simulink model "controller"  (R2024b)
settings: Solver=FixedStepAuto  StartTime=0.0  StopTime=100  FixedStep=1/10  RelTol=1e-3  EnableMultiTasking=on
undefined symbols (not defined in the file): MAX_RDB_ENGAGE_SPEED, MAX_TORQUE, MAX_TORQUE_REVERSE
libraries: arduinolib x15
settings Model: ExtModeTrigDuration=2  Creator=DAUIN-Win10  LastModifiedBy=aayan
settings SolverCC: AutoInsertRateTranBlk=on
settings OptimizationCC: EnhancedBackFolding=on  PassReuseOutputArgsAs=Individual arguments  ZeroExternalMemoryAtStartup=off  ZeroInternalMemoryAtStartup=off  MaxStackSize=64  OptimizeBlockOrder=speed  DifferentSizesBufferReuse=on  OptimizationCustomize=off  EfficientTunableParamExpr=on
settings DebuggingCC: ParameterTunabilityLossMsg=error  UnconnectedInputMsg=warning  UnconnectedOutputMsg=warning  UnconnectedLineMsg=warning
settings HardwareCC: ProdBitPerInt=16  ProdBitPerPointer=16  ProdBitPerSizeT=16  ProdBitPerPtrDiffT=16  ProdLargestAtomicFloat=None  ProdWordSize=8  ProdHWDeviceType=Atmel->AVR
settings ModelReferenceCC: EnableRefExpFcnMdlSchedulingChecks=on
settings SFSimCC: MATLABDynamicMemAlloc=off
settings RTWCC: Description=Embedded Coder  SystemTargetFile=ert.tlc  HardwareBoard=Arduino Uno  TemplateMakefile=ert_default_tmf  GenerateReport=on  Toolchain=Arduino AVR  BuildConfiguration=Faster Runs  GPUComputeCapability=3.5  DLArmComputeVersion=19.05
settings CodeAppCC: ForceParamTrailComments=on  IgnoreCustomStorageClasses=off  OperatorAnnotations=on  SimulinkDataObjDesc=on  SFDataObjDesc=on  InsertBlockDesc=on
settings ERTTargetCC: SupportVariableSizeSignals=on  ExtModeTransport=3  ExtModeStaticAlloc=on  ExtModeAutomaticAllocSize=off  ExtModeStaticAllocSize=250  ExtModeMexFile=ext_xcp  ExtModeIntrfLevel=Level2 - Open  InlinedParameterPlacement=Hierarchical

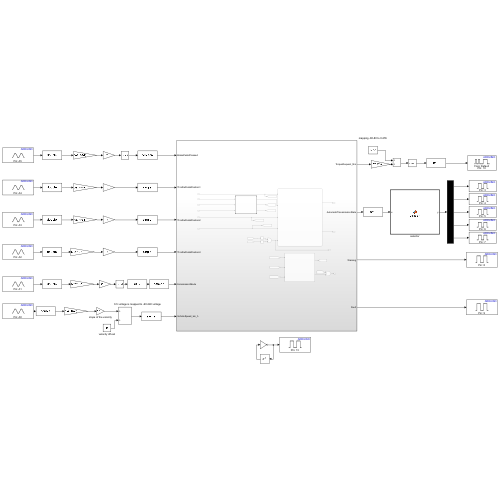
[thumbnail: Simulink's stored preview of the top-level diagram]
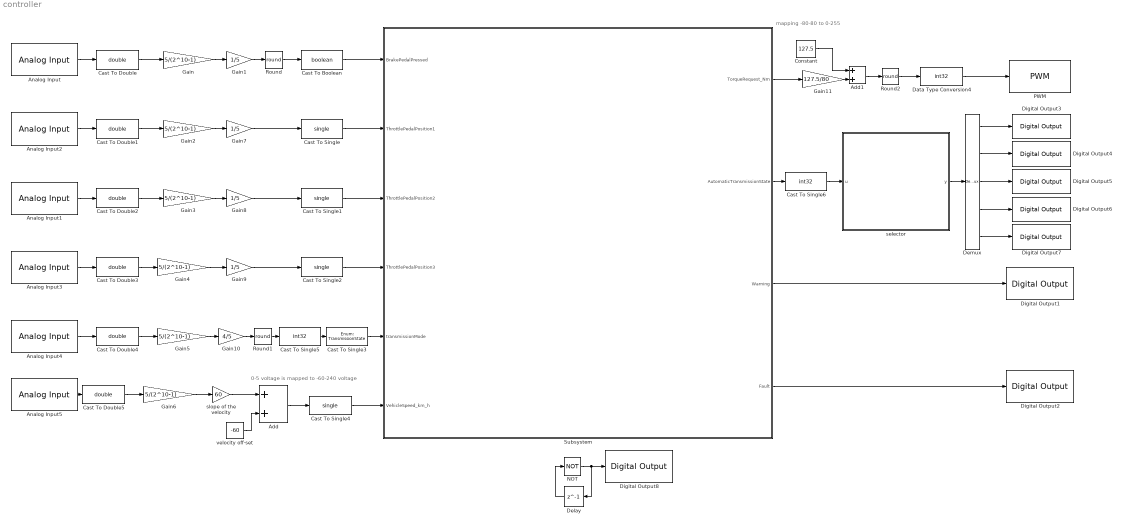
== system controller ==
  note: mapping -80-80 to 0-255
  note: 0-5 voltage is mapped to -60-240 voltage
  Add : Sum
  Add1 : Sum
  Analog Input : arduinolib/Analog Input  pinNumber=5  ReadResultsOnly=off  ConversionTriggerSource=Software  ExternalTriggerType=uint32( 0 )  OutputDataType=uint16  EnableConversionCompleteNotify=off  EnableOuputStatus=off  SampleTime=-1  blockPlatform=arduino
      settings: SourceProductName=Common
  Analog Input1 : arduinolib/Analog Input  pinNumber=3  ReadResultsOnly=off  ConversionTriggerSource=Software  ExternalTriggerType=uint32( 0 )  OutputDataType=uint16  EnableConversionCompleteNotify=off  EnableOuputStatus=off  SampleTime=-1  blockPlatform=arduino
      settings: SourceProductName=Common
  Analog Input2 : arduinolib/Analog Input  pinNumber=4  ReadResultsOnly=off  ConversionTriggerSource=Software  ExternalTriggerType=uint32( 0 )  OutputDataType=uint16  EnableConversionCompleteNotify=off  EnableOuputStatus=off  SampleTime=-1  blockPlatform=arduino
      settings: SourceProductName=Common
  Analog Input3 : arduinolib/Analog Input  pinNumber=2  ReadResultsOnly=off  ConversionTriggerSource=Software  ExternalTriggerType=uint32( 0 )  OutputDataType=uint16  EnableConversionCompleteNotify=off  EnableOuputStatus=off  SampleTime=-1  blockPlatform=arduino
      settings: SourceProductName=Common
  Analog Input4 : arduinolib/Analog Input  pinNumber=1  ReadResultsOnly=off  ConversionTriggerSource=Software  ExternalTriggerType=uint32( 0 )  OutputDataType=uint16  EnableConversionCompleteNotify=off  EnableOuputStatus=off  SampleTime=-1  blockPlatform=arduino
      settings: SourceProductName=Common
  Analog Input5 : arduinolib/Analog Input  pinNumber=0  ReadResultsOnly=off  ConversionTriggerSource=Software  ExternalTriggerType=uint32( 0 )  OutputDataType=uint16  EnableConversionCompleteNotify=off  EnableOuputStatus=off  SampleTime=-1  blockPlatform=arduino
      settings: SourceProductName=Common
  Cast To Boolean : DataTypeConversion  OutDataTypeStr=boolean  SaturateOnIntegerOverflow=off  RndMeth=Floor
  Cast To Double{,1..5} (6 alike) : DataTypeConversion  OutDataTypeStr=double  SaturateOnIntegerOverflow=off  RndMeth=Floor
  Cast To Single{,1..2,4} (4 alike) : DataTypeConversion  OutDataTypeStr=single  SaturateOnIntegerOverflow=off  RndMeth=Floor
  Cast To Single3 : DataTypeConversion  OutDataTypeStr=Enum: TransmissionState  SaturateOnIntegerOverflow=off  RndMeth=Floor
  Cast To Single5 : DataTypeConversion  OutDataTypeStr=int32  SaturateOnIntegerOverflow=off  RndMeth=Floor
  Cast To Single6 : DataTypeConversion  OutDataTypeStr=int32  SaturateOnIntegerOverflow=off  RndMeth=Floor
  Constant : Constant  Value=127.5
  Data Type Conversion4 : DataTypeConversion  OutDataTypeStr=int32  SaturateOnIntegerOverflow=off  RndMeth=Floor
  Delay : Delay  DelayLength=1  InputProcessing=Columns as channels (frame based)
  Demux : Demux  Outputs=5
  Digital Output1 : arduinolib/Digital Output  pinNumber=8  Direction=output  blockPlatform=arduino
      settings: SourceProductName=Common
  Digital Output2 : arduinolib/Digital Output  pinNumber=9  Direction=output  blockPlatform=arduino
      settings: SourceProductName=Common
  Digital Output3 : arduinolib/Digital Output  pinNumber=3  Direction=output  blockPlatform=arduino
      settings: SourceProductName=Common
  Digital Output4 : arduinolib/Digital Output  pinNumber=4  Direction=output  blockPlatform=arduino
      settings: SourceProductName=Common
  Digital Output5 : arduinolib/Digital Output  pinNumber=5  Direction=output  blockPlatform=arduino
      settings: SourceProductName=Common
  Digital Output6 : arduinolib/Digital Output  pinNumber=6  Direction=output  blockPlatform=arduino
      settings: SourceProductName=Common
  Digital Output7 : arduinolib/Digital Output  pinNumber=7  Direction=output  blockPlatform=arduino
      settings: SourceProductName=Common
  Digital Output8 : arduinolib/Digital Output  pinNumber=13  Direction=output  blockPlatform=arduino
      settings: SourceProductName=Common
  Gain{,2..6} (6 alike) : Gain  Gain=5/(2^10-1)
  Gain{1,7..9} (4 alike) : Gain  Gain=1/5
  Gain10 : Gain  Gain=4/5
  Gain11 : Gain  Gain=127.5/80
  NOT : Logic  Operator=NOT  IconShape=distinctive  AllPortsSameDT=off  OutDataTypeStr=boolean
  PWM : arduinolib/PWM  pinNumber=10  frequencyType=Default  desiredFrequency=490.2  achievableFrequency=490.2
      settings: SourceProductName=Common
  Round : Rounding  Operator=round
  Round1 : Rounding  Operator=round
  Round2 : Rounding  Operator=round
  Subsystem : Subsystem
  selector : MATLAB Function  TreatAsAtomicUnit=on
  slope of the velocity : Gain  Gain=60
  velocity off-set : Constant  Value=-60
  wires:
  Analog Input/1 -> Cast To Double/1
  Analog Input2/1 -> Cast To Double1/1
  Analog Input5/1 -> Cast To Double5/1
  Analog Input4/1 -> Cast To Double4/1
  Analog Input3/1 -> Cast To Double3/1
  Analog Input1/1 -> Cast To Double2/1
  Subsystem/1(TorqueRequest_Nm) -> Gain11/1
  Subsystem/2(AutomaticTransmissionState) -> Cast To Single6/1
  Cast To Double/1 -> Gain/1
  Gain/1 -> Gain1/1
  Gain1/1 -> Round/1
  Round/1 -> Cast To Boolean/1
  Cast To Boolean/1 -> Subsystem/1(BrakePedalPressed)
  Cast To Double1/1 -> Gain2/1
  Cast To Double2/1 -> Gain3/1
  Cast To Double3/1 -> Gain4/1
  Cast To Double4/1 -> Gain5/1
  Cast To Double5/1 -> Gain6/1
  Gain2/1 -> Gain7/1
  Gain3/1 -> Gain8/1
  Gain4/1 -> Gain9/1
  Gain5/1 -> Gain10/1
  Gain6/1 -> slope of the velocity/1
  Gain7/1 -> Cast To Single/1
  Gain8/1 -> Cast To Single1/1
  Gain9/1 -> Cast To Single2/1
  Gain10/1 -> Round1/1
  Cast To Single/1 -> Subsystem/2(ThrottlePedalPosition1)
  Cast To Single1/1 -> Subsystem/3(ThrottlePedalPosition2)
  Cast To Single2/1 -> Subsystem/4(ThrottlePedalPosition3)
  slope of the velocity/1 -> Add/1
  velocity off-set/1 -> Add/2
  Add/1 -> Cast To Single4/1
  Cast To Single3/1 -> Subsystem/5(transmissionMode)
  Cast To Single4/1 -> Subsystem/6(VehicleSpeed_km_h)
  Demux/1 -> Digital Output3/1
  Demux/2 -> Digital Output4/1
  Demux/3 -> Digital Output5/1
  Demux/4 -> Digital Output6/1
  Demux/5 -> Digital Output7/1
  Subsystem/3(Warning) -> Digital Output1/1
  Subsystem/4(Fault) -> Digital Output2/1
  Constant/1 -> Add1/1
  Gain11/1 -> Add1/2
  Add1/1 -> Round2/1
  selector/1(y) -> Demux/1
  Round2/1 -> Data Type Conversion4/1
  Data Type Conversion4/1 -> PWM/1
  Round1/1 -> Cast To Single5/1
  Cast To Single5/1 -> Cast To Single3/1
  Cast To Single6/1 -> selector/1(u)
  NOT/1 -> Digital Output8/1, Delay/1
  Delay/1 -> NOT/1

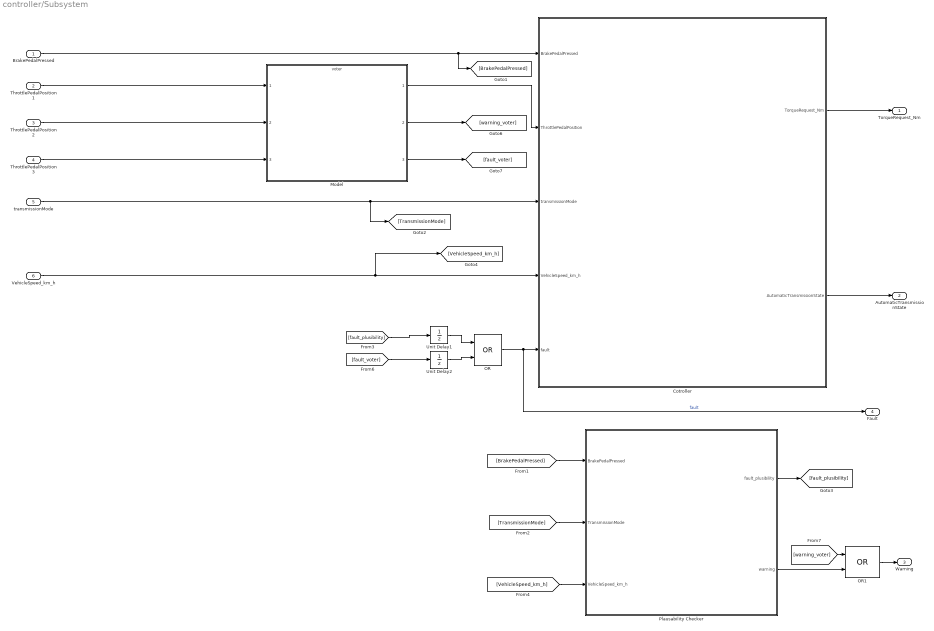
== system controller/Subsystem ==
  BrakePedalPressed : Inport
  ThrottlePedalPosition1 : Inport  Port=2
  ThrottlePedalPosition2 : Inport  Port=3
  ThrottlePedalPosition3 : Inport  Port=4
  transmissionMode : Inport  Port=5
  VehicleSpeed_km_h : Inport  Port=6
  Cotroller : Stateflow chart  TreatAsAtomicUnit=on
      settings: PortSchema="{\"entries\":[{\"content\":{\"sides\":[{\"content\":{\"connectorIds\":[\"In1\",\"In2\",\"In3\",\"In4\",\"In5\"]},\"type\":\"ConnectorPlacement.EquallySpacedRectSide\",\"uuid\":\"fa3865f3-071a-4523-b56b-dfcb7b7ff1e1\"},{\"content\":{\"connectorIds\":[\"Out2\",\"Out1\"],\"side\":\"RIGHT\"},\"type\":\"ConnectorPlacement.EquallySpacedRectSide\",\"uuid\":\"97edfdd5-6ca1-4319-83ef-4a85a5b2efa4\"},{\"content\":{\"side\":\"TOP\"},\"type\":\"ConnectorPlacement.EquallySpacedRectSide\",\"uuid\":\"bfa350c0-61e1-4051-a5a1-0c01bc7888ec\"}]},\"type\":\"ConnectorPlacement.EquallySpacedConnector\",\"uuid\":\"0069708a-38e0-4c12-a9eb-137e78633e28\"}],\"packageUris\":[\"http://schema.mathworks.com/mf0/Connector/R2020b\"],\"version\":\"1.0\"}"
  Model : ModelReference  ModelNameDialog=voter.slx  SimulationMode=Normal  ModelReferenceVersion=1.26
  OR : Logic  Operator=OR  IconShape=distinctive  AllPortsSameDT=off  OutDataTypeStr=boolean
  OR1 : Logic  Operator=OR  IconShape=distinctive  AllPortsSameDT=off  OutDataTypeStr=boolean
  Plausability Checker : Subsystem
  Unit Delay1 : UnitDelay  SampleTime=-1  HasFrameUpgradeWarning=on
  Unit Delay2 : UnitDelay  SampleTime=-1  HasFrameUpgradeWarning=on
  TorqueRequest_Nm : Outport  OutDataTypeStr=single  Unit=N*m
  AutomaticTransmissionState : Outport  Port=2  OutDataTypeStr=Enum: TransmissionState
  Warning : Outport  Port=3  OutDataTypeStr=boolean
  Fault : Outport  Port=4  OutDataTypeStr=boolean
  wires:
  BrakePedalPressed/1 -> [BrakePedalPressed], Cotroller/1(BrakePedalPressed)
  ThrottlePedalPosition1/1 -> Model/1
  ThrottlePedalPosition3/1 -> Model/3
  ThrottlePedalPosition2/1 -> Model/2
  transmissionMode/1 -> [TransmissionMode], Cotroller/3(transmissionMode)
  Model/2 -> [warning_voter]
  Plausability Checker/2(warning) -> OR1/2
  Model/3 -> [fault_voter]
  Unit Delay2/1 -> OR/2
  OR1/1 -> Warning/1
  Cotroller/1(AutomaticTransmissionState) -> AutomaticTransmissionState/1
  Unit Delay1/1 -> OR/1
  Cotroller/2(TorqueRequest_Nm) -> TorqueRequest_Nm/1
  [fault_plusibility] -> Unit Delay1/1
  [BrakePedalPressed] -> Plausability Checker/1(BrakePedalPressed)
  Plausability Checker/1(fault_plusibility) -> [fault_plusibility]
  [VehicleSpeed_km_h] -> Plausability Checker/3(VehicleSpeed_km_h)
  [fault_voter] -> Unit Delay2/1
  [warning_voter] -> OR1/1
  [TransmissionMode] -> Plausability Checker/2(TransmissionMode)
  VehicleSpeed_km_h/1 -> [VehicleSpeed_km_h], Cotroller/4(VehicleSpeed_km_h)
  Model/1 -> Cotroller/2(ThrottlePedalPosition)
  OR/1 -> Fault/1, Cotroller/5(fault)  "fault"

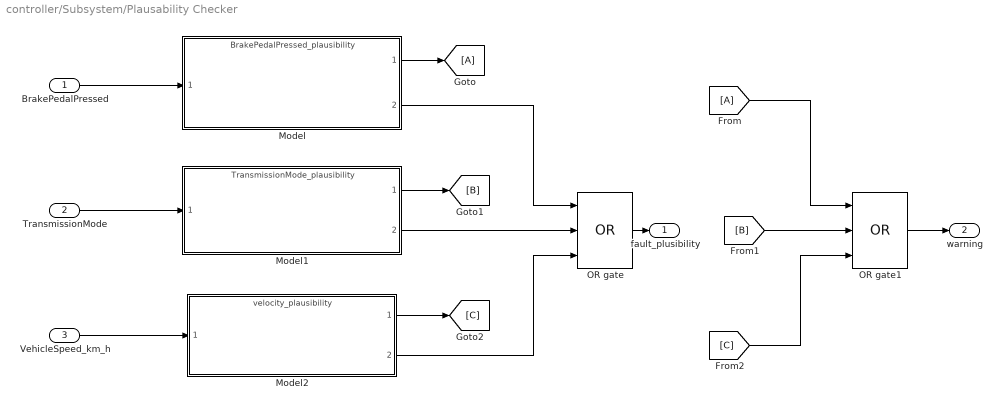
== system controller/Subsystem/Plausability Checker ==
  BrakePedalPressed : Inport
  TransmissionMode : Inport  Port=2  OutDataTypeStr=Enum: TransmissionState
  VehicleSpeed_km_h : Inport  Port=3
  From : From
  Goto : Goto
  Model : ModelReference  ModelNameDialog=BrakePedalPressed_plausibility.slx  SimulationMode=Normal  ModelReferenceVersion=1.19
  Model1 : ModelReference  ModelNameDialog=TransmissionMode_plausibility.slx  SimulationMode=Normal  ModelReferenceVersion=1.13
  Model2 : ModelReference  ModelNameDialog=velocity_plausibility.slx  SimulationMode=Normal  ModelReferenceVersion=1.14
  OR gate : Logic  Operator=OR  Inputs=3  IconShape=distinctive  AllPortsSameDT=off  OutDataTypeStr=boolean
  OR gate1 : Logic  Operator=OR  Inputs=3  IconShape=distinctive  AllPortsSameDT=off  OutDataTypeStr=boolean
  fault_plusibility : Outport  OutDataTypeStr=boolean
  warning : Outport  Port=2
  wires:
  BrakePedalPressed/1 -> Model/1
  Model/1 -> Goto/1
  TransmissionMode/1 -> Model1/1
  Model1/1 -> [B]
  Model/2 -> OR gate/1
  Model1/2 -> OR gate/2
  Model2/2 -> OR gate/3
  OR gate1/1 -> warning/1
  Model2/1 -> [C]
  From/1 -> OR gate1/1
  [B] -> OR gate1/2
  [C] -> OR gate1/3
  OR gate/1 -> fault_plusibility/1
  VehicleSpeed_km_h/1 -> Model2/1

== matlab function controller/selector ==
  data: u input; y output
function y = selector(u)

y = false(1, 5);

if u >= 0 && u <= 4
    y(u+1) = true;
end

== stateflow chart controller/Subsystem/Cotroller ==
  settings: updateMethod=DISCRETE  sampleTime=0.1
  state Park
    en:
    AutomaticTransmissionState = TransmissionState.Park;
    du:
    TorqueRequest_Nm = single(0);
  state Neutral
    en:
    AutomaticTransmissionState = TransmissionState.Neutral;
    du:
    TorqueRequest_Nm = single(0);
  state Drive
    en:
    AutomaticTransmissionState = TransmissionState.Drive;
    state ZeroTorque1
      du:
      TorqueRequest_Nm = single(0);
    state Acceleration
      du:
      TorqueRequest_Nm = single(MAX_TORQUE*(ThrottlePedalPosition));
    state StartToMove
      du:
      TorqueRequest_Nm = single(5);
    (default) -> ZeroTorque1
    ZeroTorque1 -> (junction 99) [order 1] : [BrakePedalPressed ~= 1 && VehicleSpeed_km_h  < 5 ]
    (junction 99) -> StartToMove
    (junction 94) -> ZeroTorque1
    StartToMove -> (junction 94) [order 2] : [BrakePedalPressed == 1]
    ZeroTorque1 -> Acceleration [order 2] : [(BrakePedalPressed ~= 1)]
    Acceleration -> ZeroTorque1 : [ (BrakePedalPressed == 1)]
    StartToMove -> Acceleration [order 1] : [ThrottlePedalPosition > 0 && BrakePedalPressed ~= 1]
  state Brake
    en:
    AutomaticTransmissionState = TransmissionState.Brake
    state AccelerationRegion
      du:
      TorqueRequest_Nm = single(MAX_TORQUE*(3/2)*(ThrottlePedalPosition - (1/3)));
    state ZeroTorque
      TorqueRequest_Nm = single(0);
    state DecelerationRegion
      du:
      TorqueRequest_Nm = single(-MAX_TORQUE*(1 - 3*ThrottlePedalPosition));
    (default) -> AccelerationRegion
    Brake.ZeroTorque -> AccelerationRegion : [ThrottlePedalPosition > (1/3) && BrakePedalPressed == 0]
    AccelerationRegion -> Brake.ZeroTorque [order 2] : [BrakePedalPressed == 1]
    DecelerationRegion -> AccelerationRegion [order 1] : [ (ThrottlePedalPosition >(1/3)) && BrakePedalPressed == 0]
    AccelerationRegion -> DecelerationRegion [order 1] : [ ThrottlePedalPosition < (1/3) && BrakePedalPressed == 0]
    (junction 43) -> Brake.ZeroTorque
    DecelerationRegion -> (junction 43) [order 2] : [VehicleSpeed_km_h < MAX_RDB_ENGAGE_SPEED || BrakePedalPressed == 1]
  state Reverse
    en:
    AutomaticTransmissionState = TransmissionState.Reverse;
    state Deceleration
      du:
      TorqueRequest_Nm = single(-MAX_TORQUE_REVERSE*(ThrottlePedalPosition));
    state ZeroTorque
      TorqueRequest_Nm = single(0);
    (default) -> Deceleration
    Reverse.ZeroTorque -> Deceleration : [(BrakePedalPressed == 0)]
    Deceleration -> Reverse.ZeroTorque : [(BrakePedalPressed == 1)]
  (default) -> Park
  Neutral -> Drive [order 1] : [(BrakePedalPressed == 1) && (VehicleSpeed_km_h > -5) && ((transmissionMode == TransmissionState.Drive) || (transmissionMode == TransmissionState.Brake)) && fault == 0]
  Park -> Neutral : [(BrakePedalPressed == 1) && (transmissionMode ~= TransmissionState.Park) || fault == 1]
  Drive -> Brake [order 1] : [ThrottlePedalPosition > (1/3) && (transmissionMode == TransmissionState.Brake) && fault == 0]
  Brake -> Drive : [ transmissionMode ~= TransmissionState.Brake || fault == 1]
  Drive -> Neutral [order 2] : [(transmissionMode ~= TransmissionState.Drive) && (transmissionMode ~= TransmissionState.Brake) || fault == 1]
  Neutral -> Park [order 3] : [(BrakePedalPressed == 1) && (abs(VehicleSpeed_km_h) <5) && transmissionMode == TransmissionState.Park && fault == 0]
  Neutral -> Reverse [order 2] : [(BrakePedalPressed == 1) && (VehicleSpeed_km_h < 5) && transmissionMode == TransmissionState.Reverse && fault == 0]
  Reverse -> Neutral : [transmissionMode ~= TransmissionState.Reverse || fault == 1]
  data: BrakePedalPressed input; ThrottlePedalPosition input; transmissionMode input; VehicleSpeed_km_h input; AutomaticTransmissionState output; TorqueRequest_Nm output; MAX_TORQUE parameter; MAX_TORQUE_REVERSE parameter; MAX_RDB_ENGAGE_SPEED parameter; fault input
